simulink model "Target_Control_System"  (R2021b)
settings: Solver=FixedStepDiscrete  StartTime=0.0  StopTime=5  RelTol=1e-3
PreLoadFcn:
  | RTWConfigurationCB('preloadfcn', bdroot);
PostLoadFcn:
  | load('configuration/data_struct.mat');
  | load('configuration/fluxMaps_propMotor.mat');
  | load('configuration/parameterInit_PROP.mat');
  | load('configuration/parameterInit_PUMP.mat');
  | load('configuration/parameterInit_PITCH.mat');
  | load('configuration/parameterInit_TILT.mat');
  | %load('configuration/base_workspace_signal_definition.mat');
  | %load('resolvedatastores_to_baseworkspace_for_faster_simulation.mat');
model workspace (MAT data in the model file):
  SIMULATION_OPTIONS : Simulink.Parameter (value not decoded)
  TARGET_CODE_GEN : Simulink.Parameter (value not decoded)
  TCS_SAMPLE_FREQ_HZ : Simulink.Parameter (value not decoded)
symbols that are objects in the model workspace (value not decoded): TARGET_CODE_GEN, TCS_SAMPLE_FREQ_HZ
undefined symbols (not defined in the file): A_DQ_REF_LPF_INIT__PITCH, A_DQ_REF_LPF_INIT__PROP, A_DQ_REF_LPF_INIT__PUMP, A_DQ_REF_LPF_INIT__TILT, A_OBSERVER_CONFIDENCE_INIT__PITCH, A_OBSERVER_CONFIDENCE_INIT__PROP, A_OBSERVER_CONFIDENCE_INIT__PUMP, A_OBSERVER_CONFIDENCE_INIT__TILT, ACTUATOR_MAX_ANGLE_TRIP__PITCH, ACTUATOR_MIN_ANGLE_TRIP__PITCH, ACTUATOR_POS_SENSOR_INV_DIRECTION__PITCH, ACTUATOR_POS_SENSOR_INV_DIRECTION__TILT, ACTUATOR_POS_SENSOR_OFFSET__PITCH, ACTUATOR_POS_SENSOR_OFFSET__TILT, ADC_scaler1_baseaddr_TILT, ADC_SCALER_FLOAT_TO_FIXPOINT_EXPANSION, ANGLE_ELEC_FROM_SENSOR_OFFSET_INIT__PITCH, ANGLE_ELEC_FROM_SENSOR_OFFSET_INIT__PROP, ANGLE_ELEC_FROM_SENSOR_OFFSET_INIT__PUMP, ANGLE_ELEC_FROM_SENSOR_OFFSET_INIT__TILT, AUTO_CLEAR_FAULTS_ENABLED__PITCH, AUTO_CLEAR_FAULTS_ENABLED__PROP, AUTO_CLEAR_FAULTS_ENABLED__PUMP, AUTO_CLEAR_FAULTS_ENABLED__TILT, AUTO_CLEAR_FAULTS_WAIT_TICKS__PITCH, AUTO_CLEAR_FAULTS_WAIT_TICKS__PROP, AUTO_CLEAR_FAULTS_WAIT_TICKS__PUMP, AUTO_CLEAR_FAULTS_WAIT_TICKS__TILT, AUTO_I_ZERO_IDLE_TICKS__PITCH, AUTO_I_ZERO_IDLE_TICKS__PROP, AUTO_I_ZERO_IDLE_TICKS__PUMP, AUTO_I_ZERO_IDLE_TICKS__TILT, AUTO_I_ZERO_OFFSET_IDC_THRESHOLD__PITCH, AUTO_I_ZERO_OFFSET_IDC_THRESHOLD__PROP, AUTO_I_ZERO_OFFSET_IDC_THRESHOLD__PUMP, AUTO_I_ZERO_OFFSET_IDC_THRESHOLD__TILT, AUTO_I_ZERO_OFFSET_IPH_THRESHOLD__PITCH, AUTO_I_ZERO_OFFSET_IPH_THRESHOLD__PROP, AUTO_I_ZERO_OFFSET_IPH_THRESHOLD__PUMP, AUTO_I_ZERO_OFFSET_IPH_THRESHOLD__TILT, AUTO_SENSORLESS_SWITCHOVER_DISABLE_OMEGA, AUTO_SENSORLESS_SWITCHOVER_ENABLE_OMEGA, AUTO_SENSORLESS_SWITCHOVER_MIN_CONFIDENCE, AUXILIARY_PROTECTION_UNIT_BASEADDR__TILT, blanking_max_error_omega_INIT_PITCH, blanking_max_error_omega_INIT_TILT, blanking_max_error_position_INIT_PITCH, blanking_max_error_position_INIT_TILT, BRUTE_START_I_Q_REF_RAMP_SPEED__PITCH, BRUTE_START_I_Q_REF_RAMP_SPEED__PROP, BRUTE_START_I_Q_REF_RAMP_SPEED__PUMP, BRUTE_START_I_Q_REF_RAMP_SPEED__TILT, CONTROL_LOOP_DT_INIT__PITCH, CONTROL_LOOP_DT_INIT__PROP, CONTROL_LOOP_DT_INIT__PUMP, CONTROL_LOOP_DT_INIT__TILT, CORRECTION_FILTER_SCALE__PITCH, CORRECTION_FILTER_SCALE__PROP, CORRECTION_FILTER_SCALE__PUMP, CORRECTION_FILTER_SCALE__TILT ... (+458)
libraries: simulink x178, Reusables_Lib x24
(part 33 of 47)

== system Target_Control_System/Target_Control_System/MainLoop/pitchMotor_mainLoop/mainTask_pitch/motorTaskMainFastStep()/Control Loops - Pitch/Position Controller Pitch ==
  oRampDataPos_.fRampOut : Inport
  Enable : EnablePort
  Connect PosController to CurrentController : Subsystem
  Data Store Read1 : DataStoreRead  DataStoreName=oPitch  DataStoreElements=oPitch.oMot_.oParam_.fPosition2currentPMultiplier_  IndexOptions=Index vector (dialog)  Indices=1  OutputSizes=1
  Data Store Read10 : DataStoreRead  DataStoreName=oPitch  DataStoreElements=oPitch.oMot_.oState_.oPosSensor_.oPidDataPosCtrl_.oParameter_.fLargeErrorThresholdNegative_  IndexOptions=Index vector (dialog)  Indices=1  OutputSizes=1
  Data Store Read12 : DataStoreRead  DataStoreName=oPitch  DataStoreElements=oPitch.oMot_.oState_.oPosSensor_.oPidDataPosCtrl_.oParameter_.fBlankingMaxError_  IndexOptions=Index vector (dialog)  Indices=1  OutputSizes=1
  Data Store Read14 : DataStoreRead  DataStoreName=oPitch  DataStoreElements=oPitch.oMot_.oState_.oPosSensor_.oPidDataPosCtrl_.oParameter_.fKi_  IndexOptions=Index vector (dialog)  Indices=1  OutputSizes=1
  Data Store Read15 : DataStoreRead  DataStoreName=oPitch  DataStoreElements=oPitch.oMot_.oState_.oPosSensor_.oPidDataPosCtrl_.oParameter_.fLoopDt_  IndexOptions=Index vector (dialog)  Indices=1  OutputSizes=1
  Data Store Read16 : DataStoreRead  DataStoreName=oPitch  DataStoreElements=oPitch.oMot_.oState_.oPosSensor_.oPidDataPosCtrl_.oParameter_.fIntMax_  IndexOptions=Index vector (dialog)  Indices=1  OutputSizes=1
  Data Store Read17 : DataStoreRead  DataStoreName=oPitch  DataStoreElements=oPitch.oMot_.oState_.oPosSensor_.oPidDataPosCtrl_.oParameter_.fIntMin_  IndexOptions=Index vector (dialog)  Indices=1  OutputSizes=1
  Data Store Read18 : DataStoreRead  DataStoreName=oPitch  DataStoreElements=oPitch.oMot_.oState_.oPosSensor_.oPidDataPosCtrl_.oParameter_.ipInhibitTarget_  IndexOptions=Index vector (dialog)  Indices=1  OutputSizes=1
  Data Store Read19 : DataStoreRead  DataStoreName=oPitch  DataStoreElements=oPitch.oMot_.oState_.oPosSensor_.oPidDataPosCtrl_.oParameter_.fIntegratorLeakFactor_  IndexOptions=Index vector (dialog)  Indices=1  OutputSizes=1
  Data Store Read2 : DataStoreRead  DataStoreName=oPitch  DataStoreElements=oPitch.oMot_.oParam_.fPosition2currentIMultiplier_  IndexOptions=Index vector (dialog)  Indices=1  OutputSizes=1
  Data Store Read20 : DataStoreRead  DataStoreName=oPitch  DataStoreElements=oPitch.oMot_.oState_.oPosSensor_.oPidDataPosCtrl_.oParameter_.fKd_  IndexOptions=Index vector (dialog)  Indices=1  OutputSizes=1
  Data Store Read21 : DataStoreRead  DataStoreName=oPitch  DataStoreElements=oPitch.oMot_.oState_.oPosSensor_.oPidDataPosCtrl_.oParameter_.fDMax_  IndexOptions=Index vector (dialog)  Indices=1  OutputSizes=1
  Data Store Read22 : DataStoreRead  DataStoreName=oPitch  DataStoreElements=oPitch.oMot_.oState_.oPosSensor_.oPidDataPosCtrl_.oParameter_.fDMin_  IndexOptions=Index vector (dialog)  Indices=1  OutputSizes=1
  Data Store Read23 : DataStoreRead  DataStoreName=oPitch  DataStoreElements=oPitch.oMot_.oState_.oPosSensor_.oPidDataPosCtrl_.oParameter_.fKp_  IndexOptions=Index vector (dialog)  Indices=1  OutputSizes=1
  Data Store Read24 : DataStoreRead  DataStoreName=oPitch  DataStoreElements=oPitch.oMot_.oState_.oPosSensor_.oPidDataPosCtrl_.oParameter_.fOutMin_  IndexOptions=Index vector (dialog)  Indices=1  OutputSizes=1
  Data Store Read3 : DataStoreRead  DataStoreName=oPitch  DataStoreElements=oPitch.oMot_.oState_.oPosSensor_.oPidDataPosCtrl_.oParameter_.fOutMax_  IndexOptions=Index vector (dialog)  Indices=1  OutputSizes=1
  Data Store Read4 : DataStoreRead  DataStoreName=oPitch  DataStoreElements=oPitch.oMot_.oParam_.fPosition2currentDMultiplier_  IndexOptions=Index vector (dialog)  Indices=1  OutputSizes=1
  Data Store Read5 : DataStoreRead  DataStoreName=oPitch  DataStoreElements=oPitch.oMot_.oState_.oPosSensor_.oGbx_.fCurrentOutputAngle_  IndexOptions=Index vector (dialog)  Indices=1  OutputSizes=1
  Data Store Read6 : DataStoreRead  DataStoreName=oPitch  DataStoreElements=oPitch.oMot_.oState_.oPosSensor_.oPidDataPosCtrl_.fState_  IndexOptions=Index vector (dialog)  Indices=1  OutputSizes=1
  Data Store Read7 : DataStoreRead  DataStoreName=oPitch  DataStoreElements=oPitch.oMot_.oState_.oPosSensor_.fOmegaEFromSensor_  IndexOptions=Index vector (dialog)  Indices=1  OutputSizes=1
  Data Store Read8 : DataStoreRead  DataStoreName=oPitch  DataStoreElements=oPitch.oMot_.oState_.oPosSensor_.oPidDataPosCtrl_.oParameter_.fErrorReduction_  IndexOptions=Index vector (dialog)  Indices=1  OutputSizes=1
  Data Store Read9 : DataStoreRead  DataStoreName=oPitch  DataStoreElements=oPitch.oMot_.oState_.oPosSensor_.oPidDataPosCtrl_.oParameter_.fLargeErrorThresholdPositive_  IndexOptions=Index vector (dialog)  Indices=1  OutputSizes=1
  Data Store Write : DataStoreWrite  DataStoreName=oPitch  DataStoreElements=oPitch.oMot_.oState_.oPosSensor_.oPidDataPosCtrl_.oParameter_.iLargeErrorPresent_  IndexOptions=Index vector (dialog)  Indices=1  OutputSizes=1
  Data Store Write1 : DataStoreWrite  DataStoreName=oPitch  DataStoreElements=oPitch.oMot_.oState_.oPosSensor_.oPidDataPosCtrl_.oParameter_.fITerm_  IndexOptions=Index vector (dialog)  Indices=1  OutputSizes=1
  Data Store Write2 : DataStoreWrite  DataStoreName=oPitch  DataStoreElements=oPitch.oMot_.oState_.oPosSensor_.oPidDataPosCtrl_.oParameter_.fDTerm_  IndexOptions=Index vector (dialog)  Indices=1  OutputSizes=1
  Data Store Write3 : DataStoreWrite  DataStoreName=oPitch  DataStoreElements=oPitch.oMot_.oState_.oPosSensor_.oPidDataPosCtrl_.oParameter_.fPTerm_  IndexOptions=Index vector (dialog)  Indices=1  OutputSizes=1
  Data Store Write4 : DataStoreWrite  DataStoreName=oPitch  DataStoreElements=oPitch.oMot_.oState_.oRampDataOmegaERef_.fSetpoint_  IndexOptions=Index vector (dialog)  Indices=1  OutputSizes=1
  Data Store Write5 : DataStoreWrite  DataStoreName=oPitch  DataStoreElements=oPitch.oMot_.oState_.oPosSensor_.oPidDataPosCtrl_.fState_  IndexOptions=Index vector (dialog)  Indices=1  OutputSizes=1
  Data Store Write6 : DataStoreWrite  DataStoreName=oPitch  DataStoreElements=oPitch.oMot_.oState_.fIqRefFromSpeedController_  IndexOptions=Index vector (dialog)  Indices=1  OutputSizes=1
  pid2ControllerStep(oPidDataPosCtrl)_pitch : Subsystem  TreatAsAtomicUnit=on
  oRampDataOmegaERef_.fSetpoint : Outport
  wires:
  Data Store Read6/1 -> pid2ControllerStep(oPidDataPosCtrl)_pitch/20(fpState)
  Connect PosController to CurrentController/1(fIqRefFromSpeedController) -> Data Store Write6/1
  Data Store Read1/1 -> Connect PosController to CurrentController/2(fIMultiplier)
  Data Store Read2/1 -> Connect PosController to CurrentController/1(fPMultiplier)
  Data Store Read4/1 -> Connect PosController to CurrentController/3(DMultiplier)
  pid2ControllerStep(oPidDataPosCtrl)_pitch/2(fITerm) -> Connect PosController to CurrentController/4(fITerm), Data Store Write1/1
  Data Store Read16/1 -> pid2ControllerStep(oPidDataPosCtrl)_pitch/10(fIntMax)
  pid2ControllerStep(oPidDataPosCtrl)_pitch/4(fPTerm) -> Connect PosController to CurrentController/6(fPTerm), Data Store Write3/1
  Data Store Read20/1 -> pid2ControllerStep(oPidDataPosCtrl)_pitch/13(fKd)
  Data Store Read19/1 -> pid2ControllerStep(oPidDataPosCtrl)_pitch/12(fIntegratorLeakFactor)
  Data Store Read14/1 -> pid2ControllerStep(oPidDataPosCtrl)_pitch/7(fKi)
  Data Store Read15/1 -> pid2ControllerStep(oPidDataPosCtrl)_pitch/9(fLoopDt)
  Data Store Read24/1 -> pid2ControllerStep(oPidDataPosCtrl)_pitch/19(fOutMin)
  pid2ControllerStep(oPidDataPosCtrl)_pitch/3(fDTerm) -> Data Store Write2/1, Connect PosController to CurrentController/5(fDTerm)
  Data Store Read9/1 -> pid2ControllerStep(oPidDataPosCtrl)_pitch/4(fLargeErrorThresholdPositive)
  Data Store Read21/1 -> pid2ControllerStep(oPidDataPosCtrl)_pitch/15(fDMax)
  Data Store Read3/1 -> pid2ControllerStep(oPidDataPosCtrl)_pitch/18(fOutMax)
  Data Store Read17/1 -> pid2ControllerStep(oPidDataPosCtrl)_pitch/11(fIntMin)
  Data Store Read8/1 -> pid2ControllerStep(oPidDataPosCtrl)_pitch/3(fErrorReduction)
  Data Store Read5/1 -> pid2ControllerStep(oPidDataPosCtrl)_pitch/1(fActual)
  pid2ControllerStep(oPidDataPosCtrl)_pitch/1(iLargeErrorPresent) -> Data Store Write/1
  oRampDataPos_.fRampOut/1 -> pid2ControllerStep(oPidDataPosCtrl)_pitch/2(fTarget)
  Data Store Read23/1 -> pid2ControllerStep(oPidDataPosCtrl)_pitch/17(fKp)
  Data Store Read22/1 -> pid2ControllerStep(oPidDataPosCtrl)_pitch/16(fDMin)
  Data Store Read18/1 -> pid2ControllerStep(oPidDataPosCtrl)_pitch/8(ipInhibitTarget)
  pid2ControllerStep(oPidDataPosCtrl)_pitch/5(fOutput) -> Data Store Write4/1, oRampDataOmegaERef_.fSetpoint/1
  Data Store Read12/1 -> pid2ControllerStep(oPidDataPosCtrl)_pitch/6(fBlankingMaxError)
  Data Store Read7/1 -> pid2ControllerStep(oPidDataPosCtrl)_pitch/14(fActualDt)
  pid2ControllerStep(oPidDataPosCtrl)_pitch/6(*fpState) -> Data Store Write5/1
  Data Store Read10/1 -> pid2ControllerStep(oPidDataPosCtrl)_pitch/5(fLargeErrorThresholdNegative)

== system Target_Control_System/Target_Control_System/MainLoop/pitchMotor_mainLoop/mainTask_pitch/motorTaskMainFastStep()/Control Loops - Pitch/Ramp Flux Feedforward ==
  Enable : EnablePort
  Data Store Read19 : DataStoreRead  DataStoreName=oPitch  DataStoreElements=oPitch.oMot_.oState_.oRampDataFluxFeedforwardGain_.oParam_.fTimestepS_  IndexOptions=Index vector (dialog)  Indices=1  OutputSizes=1
  Data Store Read20 : DataStoreRead  DataStoreName=oPitch  DataStoreElements=oPitch.oMot_.oState_.oRampDataFluxFeedforwardGain_.oParam_.fUpslope_  IndexOptions=Index vector (dialog)  Indices=1  OutputSizes=1
  Data Store Read21 : DataStoreRead  DataStoreName=oPitch  DataStoreElements=oPitch.oMot_.oState_.oRampDataFluxFeedforwardGain_.oParam_.fDownslope_  IndexOptions=Index vector (dialog)  Indices=1  OutputSizes=1
  Data Store Read22 : DataStoreRead  DataStoreName=oPitch  DataStoreElements=oPitch.oMot_.oState_.oRampDataFluxFeedforwardGain_.fSetpoint_  IndexOptions=Index vector (dialog)  Indices=1  OutputSizes=1
  Data Store Write10 : DataStoreWrite  DataStoreName=oPitch  DataStoreElements=oPitch.oMot_.oState_.oRampDataFluxFeedforwardGain_.fRampOutDdt_  IndexOptions=Index vector (dialog)  Indices=1  OutputSizes=1
  Data Store Write9 : DataStoreWrite  DataStoreName=oPitch  DataStoreElements=oPitch.oMot_.oState_.oRampDataFluxFeedforwardGain_.fRampOut_  IndexOptions=Index vector (dialog)  Indices=1  OutputSizes=1
  rampStep(oRampDataFluxFeedforwardGain)_pitch : Reusables_Lib/rampStep_  SystemSampleTime=-1  VariantActivationTime=update diagram  Latency=0  AutoFrameSizeCalculation=off
  wires:
  rampStep(oRampDataFluxFeedforwardGain)_pitch/1 -> Data Store Write9/1
  rampStep(oRampDataFluxFeedforwardGain)_pitch/2 -> Data Store Write10/1
  Data Store Read20/1 -> rampStep(oRampDataFluxFeedforwardGain)_pitch/2
  Data Store Read21/1 -> rampStep(oRampDataFluxFeedforwardGain)_pitch/3
  Data Store Read19/1 -> rampStep(oRampDataFluxFeedforwardGain)_pitch/4
  Data Store Read22/1 -> rampStep(oRampDataFluxFeedforwardGain)_pitch/1

== system Target_Control_System/Target_Control_System/MainLoop/pitchMotor_mainLoop/mainTask_pitch/motorTaskMainFastStep()/Control Loops - Pitch/Speed Controller Pitch ==
  oRampDataOmegaERef_.fRampOut : Inport
  Enable : EnablePort
  AND : Logic  AllPortsSameDT=off  OutDataTypeStr=boolean
  Constant : Constant  Value=245  OutDataTypeStr=int32  SampleTime=-1
  Constant1 : Constant  Value=0  OutDataTypeStr=int32  SampleTime=-1
  Data Store Read1 : DataStoreRead  DataStoreName=oPitch  DataStoreElements=oPitch.oMot_.oParam_.uiTorqueMirroringActive_  IndexOptions=Index vector (dialog)  Indices=1  OutputSizes=1
  Data Store Read2 : DataStoreRead  DataStoreName=oPitch  DataStoreElements=oPitch.oMot_.oState_.uiDriveState_  IndexOptions=Index vector (dialog)  Indices=1  OutputSizes=1
  Data Store Read3 : DataStoreRead  DataStoreName=oPitch  DataStoreElements=oPitch.oIsr_.oParam_.iUseSensorAngle_  IndexOptions=Index vector (dialog)  Indices=1  OutputSizes=1
  Enabled Subsystem : Subsystem  TreatAsAtomicUnit=on
  Enabled Subsystem1 : Subsystem  TreatAsAtomicUnit=on
  GreaterThan : RelationalOperator  Operator=>  OutDataTypeStr=boolean  RndMeth=Simplest
  Less Than : RelationalOperator  Operator=<  OutDataTypeStr=boolean  RndMeth=Simplest
  NOT : Logic  Operator=NOT  IconShape=distinctive  AllPortsSameDT=off  OutDataTypeStr=boolean
  NOT1 : Logic  Operator=NOT  AllPortsSameDT=off  OutDataTypeStr=boolean
  Set Iq Ref Pitch : Subsystem  TreatAsAtomicUnit=on
  Switch : Switch  Criteria=u2 > Threshold
  wires:
  Enabled Subsystem1/1(fIqRefFromSpeedController) -> Switch/3
  GreaterThan/1 -> Switch/2, Enabled Subsystem/Enable, NOT1/1
  Constant1/1 -> GreaterThan/2
  Data Store Read3/1 -> GreaterThan/1
  NOT1/1 -> Enabled Subsystem1/Enable
  Switch/1 -> Set Iq Ref Pitch/1(fIqRefFromSpeedController)
  Enabled Subsystem/1(fIqRefFromSpeedController) -> Switch/1
  oRampDataOmegaERef_.fRampOut/1 -> Enabled Subsystem1/1(oRampDataOmegaERef_.fRampOut), Enabled Subsystem/1(oRampDataOmegaERef_.fRampOut)
  Data Store Read2/1 -> Less Than/1
  Data Store Read1/1 -> NOT/1
  Constant/1 -> Less Than/2
  NOT/1 -> AND/1
  Less Than/1 -> AND/2
  AND/1 -> Set Iq Ref Pitch/Enable

== system Target_Control_System/Target_Control_System/MainLoop/pitchMotor_mainLoop/mainTask_pitch/motorTaskMainFastStep()/Correction Constants for Observer and Control - Pitch/1//sqrt(1+u^2) ==
  fTemp : Inport
  Add : Sum
  Constant2 : Constant  OutDataTypeStr=single  SampleTime=-1
  Constant3 : Constant  OutDataTypeStr=single  SampleTime=-1
  Divide5 : Product  Inputs=**
  Divide6 : Product  Inputs=*/
  Sqrt : Sqrt  SaturateOnIntegerOverflow=on
  Out1 : Outport
  wires:
  Divide5/1 -> Add/1
  fTemp/1 -> Divide5/1, Divide5/2
  Add/1 -> Sqrt/1
  Sqrt/1 -> Divide6/2
  Constant3/1 -> Divide6/1
  Constant2/1 -> Add/2
  Divide6/1 -> Out1/1

== system Target_Control_System/Target_Control_System/MainLoop/pitchMotor_mainLoop/mainTask_pitch/motorTaskMainFastStep()/Mechanical System - Pitch/processSensors(&oPitch) ==
  Enable : EnablePort
  Auxiliary sensor : Subsystem
  Data Store Read94 : DataStoreRead  DataStoreName=oPitch  DataStoreElements=oPitch.oMot_.oState_.oPosSensor_.eAuxiliaryPositionSensorType_  IndexOptions=Index vector (dialog)  Indices=1  OutputSizes=1
  Enumerated Constant2 : simulink/Sources/Enumerated Constant  OutDataTypeStr=Enum: EPositionSensor_t  Value=EPositionSensor_t.eNone  SampleTime=-1
  Input (motor) side sensor : Subsystem
  NotEqual : RelationalOperator  Operator=~=  OutDataTypeStr=boolean  RndMeth=Simplest
  Output (actuator) side sensor : Subsystem
  wires:
  NotEqual/1 -> Auxiliary sensor/Enable
  Enumerated Constant2/1 -> NotEqual/2
  Data Store Read94/1 -> NotEqual/1

== system Target_Control_System/Target_Control_System/MainLoop/pitchMotor_mainLoop/mainTask_pitch/motorTaskMainFastStep()/Motor Acceleration - Pitch/First filter stage ==
  function : TriggerPort  TriggerType=function-call  VariantControl=Variant
  Data Store Read : DataStoreRead  DataStoreName=mdl_pitch_fOmegaE  IndexOptions=Index vector (dialog)  Indices=1  OutputSizes=1
  Data Store Read1 : DataStoreRead  DataStoreName=oPitch  DataStoreElements=oPitch.oMot_.oState_.oMotorAccelerationFilterStage1_.afConstantsA_.h0  IndexOptions=Index vector (dialog)  Indices=1  OutputSizes=1
  Data Store Read10 : DataStoreRead  DataStoreName=oPitch  DataStoreElements=oPitch.oMot_.oState_.oMotorAccelerationFilterStage1_.afPreviousOutputs_.h1  IndexOptions=Index vector (dialog)  Indices=1  OutputSizes=1
  Data Store Read11 : DataStoreRead  DataStoreName=oPitch  DataStoreElements=oPitch.oMot_.oState_.fOmegaEPrevious_  IndexOptions=Index vector (dialog)  Indices=1  OutputSizes=1
  Data Store Read2 : DataStoreRead  DataStoreName=oPitch  DataStoreElements=oPitch.oMot_.oState_.oMotorAccelerationFilterStage1_.afConstantsA_.h1  IndexOptions=Index vector (dialog)  Indices=1  OutputSizes=1
  Data Store Read3 : DataStoreRead  DataStoreName=oPitch  DataStoreElements=oPitch.oMot_.oState_.oMotorAccelerationFilterStage1_.afConstantsA_.h2  IndexOptions=Index vector (dialog)  Indices=1  OutputSizes=1
  Data Store Read4 : DataStoreRead  DataStoreName=oPitch  DataStoreElements=oPitch.oMot_.oState_.oMotorAccelerationFilterStage1_.afConstantsB_.h0  IndexOptions=Index vector (dialog)  Indices=1  OutputSizes=1
  Data Store Read5 : DataStoreRead  DataStoreName=oPitch  DataStoreElements=oPitch.oMot_.oState_.oMotorAccelerationFilterStage1_.afConstantsB_.h1  IndexOptions=Index vector (dialog)  Indices=1  OutputSizes=1
  Data Store Read6 : DataStoreRead  DataStoreName=oPitch  DataStoreElements=oPitch.oMot_.oState_.oMotorAccelerationFilterStage1_.afConstantsB_.h2  IndexOptions=Index vector (dialog)  Indices=1  OutputSizes=1
  Data Store Read7 : DataStoreRead  DataStoreName=oPitch  DataStoreElements=oPitch.oMot_.oState_.oMotorAccelerationFilterStage1_.afPreviousInputs_.h0  IndexOptions=Index vector (dialog)  Indices=1  OutputSizes=1
  Data Store Read8 : DataStoreRead  DataStoreName=oPitch  DataStoreElements=oPitch.oMot_.oState_.oMotorAccelerationFilterStage1_.afPreviousInputs_.h1  IndexOptions=Index vector (dialog)  Indices=1  OutputSizes=1
  Data Store Read9 : DataStoreRead  DataStoreName=oPitch  DataStoreElements=oPitch.oMot_.oState_.oMotorAccelerationFilterStage1_.afPreviousOutputs_.h0  IndexOptions=Index vector (dialog)  Indices=1  OutputSizes=1
  Data Store Write1 : DataStoreWrite  DataStoreName=oPitch  DataStoreElements=oPitch.oMot_.oState_.oMotorAccelerationFilterStage1_.fFilterOutput_  IndexOptions=Index vector (dialog)  Indices=1  OutputSizes=1
  Data Store Write2 : DataStoreWrite  DataStoreName=oPitch  DataStoreElements=oPitch.oMot_.oState_.oMotorAccelerationFilterStage1_.afPreviousOutputs_.h0  IndexOptions=Index vector (dialog)  Indices=1  OutputSizes=1
  Data Store Write3 : DataStoreWrite  DataStoreName=oPitch  DataStoreElements=oPitch.oMot_.oState_.oMotorAccelerationFilterStage1_.afPreviousOutputs_.h1  IndexOptions=Index vector (dialog)  Indices=1  OutputSizes=1
  Data Store Write4 : DataStoreWrite  DataStoreName=oPitch  DataStoreElements=oPitch.oMot_.oState_.oMotorAccelerationFilterStage1_.afPreviousInputs_.h0  IndexOptions=Index vector (dialog)  Indices=1  OutputSizes=1
  Data Store Write5 : DataStoreWrite  DataStoreName=oPitch  DataStoreElements=oPitch.oMot_.oState_.oMotorAccelerationFilterStage1_.afPreviousInputs_.h1  IndexOptions=Index vector (dialog)  Indices=1  OutputSizes=1
  Subtract : Sum  Inputs=+-
  softwareIirFilterStep() : Subsystem
  wires:
  softwareIirFilterStep()/3(*afPreviousOutputs1) -> Data Store Write3/1
  Data Store Read3/1 -> softwareIirFilterStep()/7(afConstantsA2)
  Data Store Read11/1 -> Subtract/2
  Subtract/1 -> softwareIirFilterStep()/1(newInput)
  softwareIirFilterStep()/5(fFilterOutput) -> Data Store Write1/1
  Data Store Read6/1 -> softwareIirFilterStep()/4(afConstantsB2)
  Data Store Read8/1 -> softwareIirFilterStep()/9(afPreviousInputs1)
  Data Store Read/1 -> Subtract/1
  Data Store Read7/1 -> softwareIirFilterStep()/8(afPreviousInputs0)
  Data Store Read1/1 -> softwareIirFilterStep()/5(afConstantsA0)
  Data Store Read10/1 -> softwareIirFilterStep()/11(afPreviousOutputs1)
  softwareIirFilterStep()/1(*afPreviousInputs1) -> Data Store Write5/1
  softwareIirFilterStep()/4(*afPreviousOutputs0) -> Data Store Write2/1
  softwareIirFilterStep()/2(*afPreviousInputs0) -> Data Store Write4/1
  Data Store Read2/1 -> softwareIirFilterStep()/6(afConstantsA1)
  Data Store Read9/1 -> softwareIirFilterStep()/10(afPreviousOutputs0)
  Data Store Read5/1 -> softwareIirFilterStep()/3(afConstantsB1)
  Data Store Read4/1 -> softwareIirFilterStep()/2(afConstantsB0)

== system Target_Control_System/Target_Control_System/MainLoop/pitchMotor_mainLoop/mainTask_pitch/motorTaskMainFastStep()/Motor Acceleration - Pitch/Speed step ==
  function : TriggerPort  TriggerType=function-call  VariantControl=Variant
  Data Store Read : DataStoreRead  DataStoreName=mdl_pitch_fOmegaE  IndexOptions=Index vector (dialog)  Indices=1  OutputSizes=1
  Data Store Write : DataStoreWrite  DataStoreName=oPitch  DataStoreElements=oPitch.oMot_.oState_.fOmegaEPrevious_  IndexOptions=Index vector (dialog)  Indices=1  OutputSizes=1
  wires:
  Data Store Read/1 -> Data Store Write/1

== system Target_Control_System/Target_Control_System/MainLoop/pitchMotor_mainLoop/mainTask_pitch/motorTaskMainFastStep()/Observer Confidence - Pitch/Automatic switching to sensorless ==
  In1 : Inport
  Enable : EnablePort
  Data Store Read27 : DataStoreRead  DataStoreName=oPitch  DataStoreElements=oPitch.oMot_.oState_.uiSensorlessSwitchoverState_  IndexOptions=Index vector (dialog)  Indices=1  OutputSizes=1
  If : If
  "Switch to sensored? " : Subsystem  TreatAsAtomicUnit=on
  Switch to sensorless? : Subsystem  TreatAsAtomicUnit=on
  wires:
  In1/1 -> "Switch to sensored? "/1(fObserverConfidence), Switch to sensorless?/1(fObserverConfidence)
  Data Store Read27/1 -> If/1
  If/1 -> "Switch to sensored? "/Action
  If/2 -> Switch to sensorless?/Action

== system Target_Control_System/Target_Control_System/MainLoop/pitchMotor_mainLoop/mainTask_pitch/motorTaskMainFastStep()/Observer Confidence - Pitch/IIR ==
  In : Inport
  1-K : Inport  Port=2
  K : Inport  Port=3
  Product : Product  OutDataTypeStr=single  RndMeth=Zero
  Product1 : Product  RndMeth=Zero
  Sum : Sum  Inputs=|++  OutDataTypeStr=single
  Unit Delay : UnitDelay  SampleTime=-1  HasFrameUpgradeWarning=on
  Out : Outport
  wires:
  Sum/1 -> Unit Delay/1, Out/1
  Unit Delay/1 -> Product/1
  K/1 -> Product1/2
  1-K/1 -> Product/2
  Product/1 -> Sum/1
  Product1/1 -> Sum/2
  In/1 -> Product1/1

== system Target_Control_System/Target_Control_System/MainLoop/pitchMotor_mainLoop/mainTask_pitch/motorTaskMainFastStep()/Software Overcurrent Protection - Pitch/Forced_angle_overcurrent ==
  Enable : EnablePort
  Chart : Stateflow chart  TreatAsAtomicUnit=on

== system Target_Control_System/Target_Control_System/MainLoop/pitchMotor_mainLoop/mainTask_pitch/motorTaskMainFastStep()/Software Overcurrent Protection - Pitch/checkForHwOvercurrents(&oPitch) ==
  Enable : EnablePort
  "checkForHwOvercurrents " : Stateflow chart  TreatAsAtomicUnit=on
  gateDriverStatus : Subsystem  Variant=on

== system Target_Control_System/Target_Control_System/MainLoop/propMotor_mainLoop/Decimation gate for 5000 Hz Prop/motorTaskProcessExternalSetpoints(&oProp)/Subsystem1/Subsystem ==
  Enable : EnablePort
  Data Store Read68 : DataStoreRead  DataStoreName=oProp  DataStoreElements=oProp.oMot_.oParam_.fDynILimDynamicMax_  IndexOptions=Index vector (dialog)  Indices=1  OutputSizes=1
  Data Store Write19 : DataStoreWrite  DataStoreName=oProp  DataStoreElements=oProp.oMot_.oIn_.fIqSetpoint_  IndexOptions=Index vector (dialog)  Indices=1  OutputSizes=1
  wires:
  Data Store Read68/1 -> Data Store Write19/1

== system Target_Control_System/Target_Control_System/MainLoop/propMotor_mainLoop/Decimation gate for 5000 Hz Prop/motorTaskProcessExternalSetpoints(&oProp)/Subsystem2/Subsystem ==
  Enable : EnablePort
  Data Store Write19 : DataStoreWrite  DataStoreName=oProp  DataStoreElements=oProp.oMot_.oIn_.fIqSetpoint_  IndexOptions=Index vector (dialog)  Indices=1  OutputSizes=1
  const1 : Constant  Value=0.0  OutDataTypeStr=single  SampleTime=-1
  wires:
  const1/1 -> Data Store Write19/1

== system Target_Control_System/Target_Control_System/MainLoop/propMotor_mainLoop/Decimation gate for 5000 Hz Prop/motorTaskProcessExternalSetpoints(&oProp)/Subsystem3/Subsystem ==
  Enable : EnablePort
  AND : Logic  AllPortsSameDT=off  OutDataTypeStr=boolean
  AND1 : Logic  AllPortsSameDT=off  OutDataTypeStr=boolean
  Data Store Read1 : DataStoreRead  DataStoreName=oProp  DataStoreElements=oProp.oMot_.oState_.uiSpeedControllerActive_  IndexOptions=Index vector (dialog)  Indices=1  OutputSizes=1
  Data Store Read2 : DataStoreRead  DataStoreName=oProp  DataStoreElements=oProp.oMot_.oState_.oPosSensor_.iPosControlEnabled_  IndexOptions=Index vector (dialog)  Indices=1  OutputSizes=1
  Data Store Read68 : DataStoreRead  DataStoreName=oProp  DataStoreElements=oProp.oMot_.oIn_.fIqSetpoint_  IndexOptions=Index vector (dialog)  Indices=1  OutputSizes=1
  Data Store Read85 : DataStoreRead  DataStoreName=oProp  DataStoreElements=oProp.oMot_.oParam_.uiTorqueMirroringActive_  IndexOptions=Index vector (dialog)  Indices=1  OutputSizes=1
  IsNaN : RelationalOperator  Operator=isNaN  OutDataTypeStr=boolean  RndMeth=Simplest
  NOT : Logic  Operator=NOT  AllPortsSameDT=off  OutDataTypeStr=boolean
  NOT1 : Logic  Operator=NOT  AllPortsSameDT=off  OutDataTypeStr=boolean
  NOT2 : Logic  Operator=NOT  AllPortsSameDT=off  OutDataTypeStr=boolean
  OR : Logic  Operator=OR  AllPortsSameDT=off  OutDataTypeStr=boolean
  Subsystem : Subsystem
  wires:
  AND1/1 -> Subsystem/Enable
  Data Store Read85/1 -> OR/1
  Data Store Read1/1 -> NOT/1
  AND/1 -> OR/2
  NOT/1 -> AND/1
  Data Store Read2/1 -> NOT1/1
  NOT1/1 -> AND/2
  OR/1 -> AND1/1
  Data Store Read68/1 -> IsNaN/1
  IsNaN/1 -> NOT2/1
  NOT2/1 -> AND1/2

== system Target_Control_System/Target_Control_System/MainLoop/propMotor_mainLoop/Decimation gate for 5000 Hz Prop/motorTaskProcessExternalSetpoints(&oProp)/Subsystem3/Subsystem1 ==
  Enable : EnablePort
  AND1 : Logic  Operator=OR  AllPortsSameDT=off  OutDataTypeStr=boolean
  Data Store Read1 : DataStoreRead  DataStoreName=oProp  DataStoreElements=oProp.oMot_.oIn_.fIdSetpoint_  IndexOptions=Index vector (dialog)  Indices=1  OutputSizes=1
  IsNaN : RelationalOperator  Operator=isNaN  OutDataTypeStr=boolean  RndMeth=Simplest
  IsNaN1 : RelationalOperator  Operator=isInf  OutDataTypeStr=boolean  RndMeth=Simplest
  NOT1 : Logic  Operator=NOT  AllPortsSameDT=off  OutDataTypeStr=boolean
  Subsystem : Subsystem
  wires:
  NOT1/1 -> AND1/1
  Data Store Read1/1 -> IsNaN1/1, Subsystem/1(Input), IsNaN/1
  IsNaN1/1 -> AND1/2
  IsNaN/1 -> NOT1/1
  AND1/1 -> Subsystem/Enable

== system Target_Control_System/Target_Control_System/MainLoop/propMotor_mainLoop/Decimation gate for 5000 Hz Prop/motorTaskProcessExternalSetpoints(&oProp)/Subsystem3/Subsystem2 ==
  Enable : EnablePort
  AND1 : Logic  Inputs=3  AllPortsSameDT=off  OutDataTypeStr=boolean
  Data Store Read1 : DataStoreRead  DataStoreName=oProp  DataStoreElements=oProp.oMot_.oState_.oPosSensor_.iPosControlEnabled_  IndexOptions=Index vector (dialog)  Indices=1  OutputSizes=1
  Data Store Read2 : DataStoreRead  DataStoreName=oProp  DataStoreElements=oProp.oMot_.oParam_.uiAutomaticFanControlMode_  IndexOptions=Index vector (dialog)  Indices=1  OutputSizes=1
  Data Store Read85 : DataStoreRead  DataStoreName=oProp  DataStoreElements=oProp.oMot_.oState_.uiDriveState_  IndexOptions=Index vector (dialog)  Indices=1  OutputSizes=1
  Equal13 : RelationalOperator  Operator=~=  OutDataTypeStr=boolean  RndMeth=Simplest
  NOT1 : Logic  Operator=NOT  AllPortsSameDT=off  OutDataTypeStr=boolean
  NOT2 : Logic  Operator=NOT  AllPortsSameDT=off  OutDataTypeStr=boolean
  Subsystem : Subsystem
  const17 : Constant  Value=228  OutDataTypeStr=uint32  SampleTime=-1
  wires:
  Data Store Read2/1 -> NOT2/1
  NOT2/1 -> AND1/2
  const17/1 -> Equal13/1
  Data Store Read85/1 -> Equal13/2
  Equal13/1 -> AND1/3
  NOT1/1 -> AND1/1
  Data Store Read1/1 -> NOT1/1
  AND1/1 -> Subsystem/Enable

== system Target_Control_System/Target_Control_System/MainLoop/propMotor_mainLoop/Decimation gate for 5000 Hz Prop/motorTaskProcessExternalSetpoints(&oProp)/Subsystem3/Subsystem3 ==
  Enable : EnablePort
  AND : Logic  Operator=OR  AllPortsSameDT=off  OutDataTypeStr=boolean
  AND1 : Logic  Inputs=3  AllPortsSameDT=off  OutDataTypeStr=boolean
  Data Store Read1 : DataStoreRead  DataStoreName=oProp  DataStoreElements=oProp.oMot_.oState_.oPosSensor_.iPosControlEnabled_  IndexOptions=Index vector (dialog)  Indices=1  OutputSizes=1
  Data Store Read68 : DataStoreRead  DataStoreName=oProp  DataStoreElements=oProp.oMot_.oIn_.fPosSetpoint_  IndexOptions=Index vector (dialog)  Indices=1  OutputSizes=1
  Data Store Read85 : DataStoreRead  DataStoreName=oProp  DataStoreElements=oProp.oMot_.oState_.uiDriveState_  IndexOptions=Index vector (dialog)  Indices=1  OutputSizes=1
  Equal1 : RelationalOperator  Operator=~=  OutDataTypeStr=boolean  RndMeth=Simplest
  Equal13 : RelationalOperator  Operator===  OutDataTypeStr=boolean  RndMeth=Simplest
  IsNaN : RelationalOperator  Operator=isNaN  OutDataTypeStr=boolean  RndMeth=Simplest
  NOT2 : Logic  Operator=NOT  AllPortsSameDT=off  OutDataTypeStr=boolean
  Subsystem : Subsystem
  const1 : Constant  Value=202  OutDataTypeStr=uint32  SampleTime=-1
  const17 : Constant  Value=228  OutDataTypeStr=uint32  SampleTime=-1
  wires:
  NOT2/1 -> AND1/3
  const1/1 -> Equal1/2
  Equal1/1 -> AND1/2
  const17/1 -> Equal13/1
  Data Store Read85/1 -> Equal1/1, Equal13/2
  Equal13/1 -> AND/2
  AND/1 -> AND1/1
  Data Store Read1/1 -> AND/1
  IsNaN/1 -> NOT2/1
  Data Store Read68/1 -> IsNaN/1
  AND1/1 -> Subsystem/Enable

== system Target_Control_System/Target_Control_System/MainLoop/propMotor_mainLoop/Decimation gate for 5000 Hz Prop/motorTaskProcessExternalSetpoints(&oProp)/Subsystem3/Subsystem4 ==
  Enable : EnablePort
  Data Store Write1 : DataStoreWrite  DataStoreName=oProp  DataStoreElements=oProp.oMot_.oState_.fIdExternalSetpoint_  IndexOptions=Index vector (dialog)  Indices=1  OutputSizes=1
  Data Store Write19 : DataStoreWrite  DataStoreName=oProp  DataStoreElements=oProp.oMot_.oState_.oRampDataIdRef_.fSetpoint_  IndexOptions=Index vector (dialog)  Indices=1  OutputSizes=1
  const1 : Constant  Value=0.0  OutDataTypeStr=single  SampleTime=-1
  wires:
  const1/1 -> Data Store Write19/1, Data Store Write1/1

== system Target_Control_System/Target_Control_System/MainLoop/propMotor_mainLoop/motorTaskMainFastStep(&oProp)/Control Loops - Prop/Sim Options Prop Id Variant Subsystem/Sim Options 0 Prop Id Subsystem ==
  Data Store Read1 : DataStoreRead  DataStoreName=oProp  DataStoreElements=oProp.oMot_.oState_.oRampDataIdRef_.fSetpoint_  IndexOptions=Index vector (dialog)  Indices=1  OutputSizes=1
  Scope : Scope
  Out1 : Outport
  wires:
  Data Store Read1/1 -> Out1/1, Scope/1

== system Target_Control_System/Target_Control_System/MainLoop/propMotor_mainLoop/motorTaskMainFastStep(&oProp)/Control Loops - Prop/Sim Options Prop Id Variant Subsystem/Sim Options 1 Prop Iq Subsystem ==
  Constant : Constant  Value=0  OutDataTypeStr=single  SampleTime=-1
  Constant1 : Constant  OutDataTypeStr=uint32  SampleTime=-1
  Data Store Write : DataStoreWrite  DataStoreName=oProp  DataStoreElements=oProp.oMot_.oState_.oRampDataIdRef_.fSetpoint_  IndexOptions=Index vector (dialog)  Indices=1  OutputSizes=1
  Data Store Write2 : DataStoreWrite  DataStoreName=oProp  DataStoreElements=oProp.oMot_.oOut_.uiCurrentControllerActive_  IndexOptions=Index vector (dialog)  Indices=1  OutputSizes=1
  Out1 : Outport
  wires:
  Constant1/1 -> Data Store Write2/1
  Constant/1 -> Out1/1, Data Store Write/1

== system Target_Control_System/Target_Control_System/MainLoop/propMotor_mainLoop/motorTaskMainFastStep(&oProp)/Control Loops - Prop/Sim Options Prop Iq Variant Subsystem/Sim Options 0 Prop Iq Subsystem ==
  Data Store Read1 : DataStoreRead  DataStoreName=oProp  DataStoreElements=oProp.oMot_.oState_.oRampDataIqRef_.fSetpoint_  IndexOptions=Index vector (dialog)  Indices=1  OutputSizes=1
  Scope : Scope
  Out1 : Outport
  wires:
  Data Store Read1/1 -> Out1/1, Scope/1

== system Target_Control_System/Target_Control_System/MainLoop/propMotor_mainLoop/motorTaskMainFastStep(&oProp)/Control Loops - Prop/Sim Options Prop Iq Variant Subsystem/Sim Options 1 Prop Iq Subsystem ==
  Constant : Constant  Value=300  OutDataTypeStr=single
  Constant1 : Constant  OutDataTypeStr=uint32  SampleTime=-1
  Data Store Write : DataStoreWrite  DataStoreName=oProp  DataStoreElements=oProp.oMot_.oState_.oRampDataIqRef_.fSetpoint_  IndexOptions=Index vector (dialog)  Indices=1  OutputSizes=1
  Data Store Write2 : DataStoreWrite  DataStoreName=oProp  DataStoreElements=oProp.oMot_.oOut_.uiCurrentControllerActive_  IndexOptions=Index vector (dialog)  Indices=1  OutputSizes=1
  Out1 : Outport
  wires:
  Constant1/1 -> Data Store Write2/1
  Constant/1 -> Out1/1, Data Store Write/1

== system Target_Control_System/Target_Control_System/MainLoop/propMotor_mainLoop/motorTaskMainFastStep(&oProp)/Control Loops - Prop/Subsystem2/Subsystem ==
  fFluxWeakeningModulationTarget_ : Inport
  fModulationIndexSquared : Inport  Port=2
  fFluxWeakeningState_ : Inport  Port=3
  fIntControlLoopDt_ : Inport  Port=4
  Enable : EnablePort
  Add : Sum  Inputs=|++
  Add3 : Sum  Inputs=-+
  Constant4 : Constant  Value=0  OutDataTypeStr=single  SampleTime=-1
  Data Store Read94 : DataStoreRead  DataStoreName=oProp  DataStoreElements=oProp.oMot_.oParam_.fFluxWeakeningUpRampGain_  IndexOptions=Index vector (dialog)  Indices=1  OutputSizes=1
  Data Store Read96 : DataStoreRead  DataStoreName=oProp  DataStoreElements=oProp.oMot_.oParam_.fFluxWeakeningMaxCurrent_  IndexOptions=Index vector (dialog)  Indices=1  OutputSizes=1
  Display : Display
  Product : Product
  Product3 : Product
  Saturation Dynamic : simulink/Discontinuities/Saturation Dynamic  OutMin=[]  OutMax=[]  OutDataTypeStr=Inherit: Same as second input  OutDataType=fixdt(1, 16)  OutScaling=2^-10  DoSatur=off
  Out1 : Outport
  wires:
  Constant4/1 -> Saturation Dynamic/3
  Add/1 -> Saturation Dynamic/2
  Product/1 -> Add/1
  Product3/1 -> Product/1
  fIntControlLoopDt_/1 -> Product/2
  fFluxWeakeningState_/1 -> Add/2
  Data Store Read96/1 -> Display/1, Saturation Dynamic/1
  Add3/1 -> Product3/1  "fDelta"
  fFluxWeakeningModulationTarget_/1 -> Add3/1
  fModulationIndexSquared/1 -> Add3/2
  Saturation Dynamic/1 -> Out1/1
  Data Store Read94/1 -> Product3/2

== system Target_Control_System/Target_Control_System/MainLoop/propMotor_mainLoop/motorTaskMainFastStep(&oProp)/Control Loops - Prop/Subsystem2/Subsystem1 ==
  fFluxWeakeningDownRamp_ : Inport
  fIntControlLoopDt_ : Inport  Port=2
  fFluxWeakeningState_ : Inport  Port=3
  Enable : EnablePort
  Add13 : Sum  Inputs=-+
  Constant4 : Constant  Value=0  OutDataTypeStr=single  SampleTime=-1
  Product2 : Product
  Switch9 : Switch  Criteria=u2 > Threshold
  Out1 : Outport
  wires:
  Constant4/1 -> Switch9/3
  Add13/1 -> Switch9/1
  Switch9/1 -> Out1/1
  fFluxWeakeningState_/1 -> Add13/2, Switch9/2
  fFluxWeakeningDownRamp_/1 -> Product2/1
  Product2/1 -> Add13/1
  fIntControlLoopDt_/1 -> Product2/2

== system Target_Control_System/Target_Control_System/MainLoop/propMotor_mainLoop/motorTaskMainFastStep(&oProp)/Correction Constants for Observer and Control - Prop/Variant Subsystem/Simulation Subsystem ==
  In1 : Inport
  Gain6 : Gain  Gain=1/(6000*2*pi)
  Out1 : Outport
  wires:
  Gain6/1 -> Out1/1
  In1/1 -> Gain6/1

== system Target_Control_System/Target_Control_System/MainLoop/propMotor_mainLoop/motorTaskMainFastStep(&oProp)/Correction Constants for Observer and Control - Prop/Variant Subsystem/Target Code Gen Subsystem ==
  In1 : Inport
  Data Store Read9 : DataStoreRead  DataStoreName=oProp  DataStoreElements=oProp.oMot_.oParam_.fUphaseIirFLpfRads_  IndexOptions=Index vector (dialog)  Indices=1  OutputSizes=1
  Divide2 : Product  Inputs=*/
  Out1 : Outport
  wires:
  In1/1 -> Divide2/1
  Data Store Read9/1 -> Divide2/2
  Divide2/1 -> Out1/1

== system Target_Control_System/Target_Control_System/MainLoop/propMotor_mainLoop/motorTaskMainFastStep(&oProp)/PWM for Simulation/Subsystem1/Subsystem ==
  Enable : EnablePort
  Bus Creator2 : BusCreator  Inputs=3
  Data Store Read2 : DataStoreRead  DataStoreName=oProp  DataStoreElements=oProp.oMot_.oOut_.uiPwmDutyTicksFromMainA_  IndexOptions=Index vector (dialog)  Indices=1  OutputSizes=1
  Data Store Read3 : DataStoreRead  DataStoreName=oProp  DataStoreElements=oProp.oMot_.oOut_.uiPwmDutyTicksFromMainB_  IndexOptions=Index vector (dialog)  Indices=1  OutputSizes=1
  Data Store Read5 : DataStoreRead  DataStoreName=oProp  DataStoreElements=oProp.oMot_.oOut_.uiPwmDutyTicksFromMainC_  IndexOptions=Index vector (dialog)  Indices=1  OutputSizes=1
  propMotor_PWMticks : Outport
  wires:
  Data Store Read3/1 -> Bus Creator2/2  "Bticks"
  Data Store Read5/1 -> Bus Creator2/3  "Cticks"
  Bus Creator2/1 -> propMotor_PWMticks/1
  Data Store Read2/1 -> Bus Creator2/1  "Aticks"

== system Target_Control_System/Target_Control_System/MainLoop/pumpMotor_mainLoop/Decimation gate for 5000 Hz Pump/motorTaskProcessExternalSetpoints(&oPump)/Subsystem1/Subsystem ==
  Enable : EnablePort
  Data Store Read68 : DataStoreRead  DataStoreName=oPump  DataStoreElements=oPump.oMot_.oParam_.fDynILimDynamicMax_  IndexOptions=Index vector (dialog)  Indices=1  OutputSizes=1
  Data Store Write19 : DataStoreWrite  DataStoreName=oPump  DataStoreElements=oPump.oMot_.oIn_.fIqSetpoint_  IndexOptions=Index vector (dialog)  Indices=1  OutputSizes=1
  wires:
  Data Store Read68/1 -> Data Store Write19/1

== system Target_Control_System/Target_Control_System/MainLoop/pumpMotor_mainLoop/Decimation gate for 5000 Hz Pump/motorTaskProcessExternalSetpoints(&oPump)/Subsystem2/Subsystem ==
  Enable : EnablePort
  Data Store Write19 : DataStoreWrite  DataStoreName=oPump  DataStoreElements=oPump.oMot_.oIn_.fIqSetpoint_  IndexOptions=Index vector (dialog)  Indices=1  OutputSizes=1
  const1 : Constant  Value=0.0  OutDataTypeStr=single  SampleTime=-1
  wires:
  const1/1 -> Data Store Write19/1

== system Target_Control_System/Target_Control_System/MainLoop/pumpMotor_mainLoop/Decimation gate for 5000 Hz Pump/motorTaskProcessExternalSetpoints(&oPump)/Subsystem3/Subsystem ==
  Enable : EnablePort
  AND : Logic  AllPortsSameDT=off  OutDataTypeStr=boolean
  AND1 : Logic  AllPortsSameDT=off  OutDataTypeStr=boolean
  Data Store Read1 : DataStoreRead  DataStoreName=oPump  DataStoreElements=oPump.oMot_.oState_.uiSpeedControllerActive_  IndexOptions=Index vector (dialog)  Indices=1  OutputSizes=1
  Data Store Read2 : DataStoreRead  DataStoreName=oPump  DataStoreElements=oPump.oMot_.oState_.oPosSensor_.iPosControlEnabled_  IndexOptions=Index vector (dialog)  Indices=1  OutputSizes=1
  Data Store Read68 : DataStoreRead  DataStoreName=oPump  DataStoreElements=oPump.oMot_.oIn_.fIqSetpoint_  IndexOptions=Index vector (dialog)  Indices=1  OutputSizes=1
  Data Store Read85 : DataStoreRead  DataStoreName=oPump  DataStoreElements=oPump.oMot_.oParam_.uiTorqueMirroringActive_  IndexOptions=Index vector (dialog)  Indices=1  OutputSizes=1
  IsNaN : RelationalOperator  Operator=isNaN  OutDataTypeStr=boolean  RndMeth=Simplest
  NOT : Logic  Operator=NOT  AllPortsSameDT=off  OutDataTypeStr=boolean
  NOT1 : Logic  Operator=NOT  AllPortsSameDT=off  OutDataTypeStr=boolean
  NOT2 : Logic  Operator=NOT  AllPortsSameDT=off  OutDataTypeStr=boolean
  OR : Logic  Operator=OR  AllPortsSameDT=off  OutDataTypeStr=boolean
  Subsystem : Subsystem
  wires:
  AND1/1 -> Subsystem/Enable
  Data Store Read85/1 -> OR/1
  Data Store Read1/1 -> NOT/1
  AND/1 -> OR/2
  NOT/1 -> AND/1
  Data Store Read2/1 -> NOT1/1
  NOT1/1 -> AND/2
  OR/1 -> AND1/1
  Data Store Read68/1 -> IsNaN/1
  IsNaN/1 -> NOT2/1
  NOT2/1 -> AND1/2

== system Target_Control_System/Target_Control_System/MainLoop/pumpMotor_mainLoop/Decimation gate for 5000 Hz Pump/motorTaskProcessExternalSetpoints(&oPump)/Subsystem3/Subsystem1 ==
  Enable : EnablePort
  AND1 : Logic  Operator=OR  AllPortsSameDT=off  OutDataTypeStr=boolean
  Data Store Read1 : DataStoreRead  DataStoreName=oPump  DataStoreElements=oPump.oMot_.oIn_.fIdSetpoint_  IndexOptions=Index vector (dialog)  Indices=1  OutputSizes=1
  IsNaN : RelationalOperator  Operator=isNaN  OutDataTypeStr=boolean  RndMeth=Simplest
  IsNaN1 : RelationalOperator  Operator=isInf  OutDataTypeStr=boolean  RndMeth=Simplest
  NOT1 : Logic  Operator=NOT  AllPortsSameDT=off  OutDataTypeStr=boolean
  Subsystem : Subsystem
  wires:
  NOT1/1 -> AND1/1
  Data Store Read1/1 -> IsNaN1/1, Subsystem/1(Input), IsNaN/1
  IsNaN1/1 -> AND1/2
  IsNaN/1 -> NOT1/1
  AND1/1 -> Subsystem/Enable

== system Target_Control_System/Target_Control_System/MainLoop/pumpMotor_mainLoop/Decimation gate for 5000 Hz Pump/motorTaskProcessExternalSetpoints(&oPump)/Subsystem3/Subsystem2 ==
  Enable : EnablePort
  AND1 : Logic  Inputs=3  AllPortsSameDT=off  OutDataTypeStr=boolean
  Data Store Read1 : DataStoreRead  DataStoreName=oPump  DataStoreElements=oPump.oMot_.oState_.oPosSensor_.iPosControlEnabled_  IndexOptions=Index vector (dialog)  Indices=1  OutputSizes=1
  Data Store Read2 : DataStoreRead  DataStoreName=oPump  DataStoreElements=oPump.oMot_.oParam_.uiAutomaticFanControlMode_  IndexOptions=Index vector (dialog)  Indices=1  OutputSizes=1
  Data Store Read85 : DataStoreRead  DataStoreName=oPump  DataStoreElements=oPump.oMot_.oState_.uiDriveState_  IndexOptions=Index vector (dialog)  Indices=1  OutputSizes=1
  Equal13 : RelationalOperator  Operator=~=  OutDataTypeStr=boolean  RndMeth=Simplest
  NOT1 : Logic  Operator=NOT  AllPortsSameDT=off  OutDataTypeStr=boolean
  NOT2 : Logic  Operator=NOT  AllPortsSameDT=off  OutDataTypeStr=boolean
  Subsystem : Subsystem
  const17 : Constant  Value=228  OutDataTypeStr=uint32  SampleTime=-1
  wires:
  Data Store Read2/1 -> NOT2/1
  NOT2/1 -> AND1/2
  const17/1 -> Equal13/1
  Data Store Read85/1 -> Equal13/2
  Equal13/1 -> AND1/3
  NOT1/1 -> AND1/1
  Data Store Read1/1 -> NOT1/1
  AND1/1 -> Subsystem/Enable

== system Target_Control_System/Target_Control_System/MainLoop/pumpMotor_mainLoop/Decimation gate for 5000 Hz Pump/motorTaskProcessExternalSetpoints(&oPump)/Subsystem3/Subsystem3 ==
  Enable : EnablePort
  AND : Logic  Operator=OR  AllPortsSameDT=off  OutDataTypeStr=boolean
  AND1 : Logic  Inputs=3  AllPortsSameDT=off  OutDataTypeStr=boolean
  Data Store Read1 : DataStoreRead  DataStoreName=oPump  DataStoreElements=oPump.oMot_.oState_.oPosSensor_.iPosControlEnabled_  IndexOptions=Index vector (dialog)  Indices=1  OutputSizes=1
  Data Store Read68 : DataStoreRead  DataStoreName=oPump  DataStoreElements=oPump.oMot_.oIn_.fPosSetpoint_  IndexOptions=Index vector (dialog)  Indices=1  OutputSizes=1
  Data Store Read85 : DataStoreRead  DataStoreName=oPump  DataStoreElements=oPump.oMot_.oState_.uiDriveState_  IndexOptions=Index vector (dialog)  Indices=1  OutputSizes=1
  Equal1 : RelationalOperator  Operator=~=  OutDataTypeStr=boolean  RndMeth=Simplest
  Equal13 : RelationalOperator  Operator===  OutDataTypeStr=boolean  RndMeth=Simplest
  IsNaN : RelationalOperator  Operator=isNaN  OutDataTypeStr=boolean  RndMeth=Simplest
  NOT2 : Logic  Operator=NOT  AllPortsSameDT=off  OutDataTypeStr=boolean
  Subsystem : Subsystem
  const1 : Constant  Value=202  OutDataTypeStr=uint32  SampleTime=-1
  const17 : Constant  Value=228  OutDataTypeStr=uint32  SampleTime=-1
  wires:
  NOT2/1 -> AND1/3
  const1/1 -> Equal1/2
  Equal1/1 -> AND1/2
  const17/1 -> Equal13/1
  Data Store Read85/1 -> Equal1/1, Equal13/2
  Equal13/1 -> AND/2
  AND/1 -> AND1/1
  Data Store Read1/1 -> AND/1
  IsNaN/1 -> NOT2/1
  Data Store Read68/1 -> IsNaN/1
  AND1/1 -> Subsystem/Enable

== system Target_Control_System/Target_Control_System/MainLoop/pumpMotor_mainLoop/Decimation gate for 5000 Hz Pump/motorTaskProcessExternalSetpoints(&oPump)/Subsystem3/Subsystem4 ==
  Enable : EnablePort
  Data Store Write1 : DataStoreWrite  DataStoreName=oPump  DataStoreElements=oPump.oMot_.oState_.fIdExternalSetpoint_  IndexOptions=Index vector (dialog)  Indices=1  OutputSizes=1
  Data Store Write19 : DataStoreWrite  DataStoreName=oPump  DataStoreElements=oPump.oMot_.oState_.oRampDataIdRef_.fSetpoint_  IndexOptions=Index vector (dialog)  Indices=1  OutputSizes=1
  const1 : Constant  Value=0.0  OutDataTypeStr=single  SampleTime=-1
  wires:
  const1/1 -> Data Store Write19/1, Data Store Write1/1

== system Target_Control_System/Target_Control_System/MainLoop/pumpMotor_mainLoop/motorTaskMainFastStep(&oPump)/Control Loops - Pump/Sim Options Prop Id Variant Subsystem/Sim Options 0 Prop Id Subsystem ==
  Data Store Read88 : DataStoreRead  DataStoreName=oPump  DataStoreElements=oPump.oMot_.oState_.oRampDataIdRef_.fSetpoint_  IndexOptions=Index vector (dialog)  Indices=1  OutputSizes=1
  Out1 : Outport
  wires:
  Data Store Read88/1 -> Out1/1

== system Target_Control_System/Target_Control_System/MainLoop/pumpMotor_mainLoop/motorTaskMainFastStep(&oPump)/Control Loops - Pump/Sim Options Prop Id Variant Subsystem/Sim Options 1 Prop Id Subsystem ==
  Constant : Constant  Value=0  OutDataTypeStr=single  SampleTime=-1
  Constant1 : Constant  OutDataTypeStr=uint32  SampleTime=-1
  Data Store Write : DataStoreWrite  DataStoreName=oPump  DataStoreElements=oPump.oMot_.oState_.oRampDataIdRef_.fSetpoint_  IndexOptions=Index vector (dialog)  Indices=1  OutputSizes=1
  Data Store Write2 : DataStoreWrite  DataStoreName=oPump  DataStoreElements=oPump.oMot_.oOut_.uiCurrentControllerActive_  IndexOptions=Index vector (dialog)  Indices=1  OutputSizes=1
  Out1 : Outport
  wires:
  Constant1/1 -> Data Store Write2/1
  Constant/1 -> Out1/1, Data Store Write/1

== system Target_Control_System/Target_Control_System/MainLoop/pumpMotor_mainLoop/motorTaskMainFastStep(&oPump)/Control Loops - Pump/Sim Options Pump Iq Variant Subsystem/Sim Options 0 Pump Iq Subsystem ==
  Data Store Read88 : DataStoreRead  DataStoreName=oPump  DataStoreElements=oPump.oMot_.oState_.oRampDataIqRef_.fSetpoint_  IndexOptions=Index vector (dialog)  Indices=1  OutputSizes=1
  fSetpoint_ : Outport
  wires:
  Data Store Read88/1 -> fSetpoint_/1

== system Target_Control_System/Target_Control_System/MainLoop/pumpMotor_mainLoop/motorTaskMainFastStep(&oPump)/Control Loops - Pump/Sim Options Pump Iq Variant Subsystem/Sim Options 1 Pump Iq Subsystem ==
  Constant : Constant  Value=1.5  OutDataTypeStr=single
  Constant1 : Constant  OutDataTypeStr=uint32  SampleTime=-1
  Data Store Write : DataStoreWrite  DataStoreName=oPump  DataStoreElements=oPump.oMot_.oState_.oRampDataIqRef_.fSetpoint_  IndexOptions=Index vector (dialog)  Indices=1  OutputSizes=1
  Data Store Write2 : DataStoreWrite  DataStoreName=oPump  DataStoreElements=oPump.oMot_.oOut_.uiCurrentControllerActive_  IndexOptions=Index vector (dialog)  Indices=1  OutputSizes=1
  fSetpoint_ : Outport
  wires:
  Constant1/1 -> Data Store Write2/1
  Constant/1 -> fSetpoint_/1, Data Store Write/1

== system Target_Control_System/Target_Control_System/MainLoop/pumpMotor_mainLoop/motorTaskMainFastStep(&oPump)/Control Loops - Pump/Sim Options Pump OmegaERef Variant Subsystem/Sim Options 0 Pump OmegaE Subsystem ==
  Data Store Read88 : DataStoreRead  DataStoreName=oPump  DataStoreElements=oPump.oMot_.oState_.oRampDataOmegaERef_.fSetpoint_  IndexOptions=Index vector (dialog)  Indices=1  OutputSizes=1
  Out1 : Outport
  wires:
  Data Store Read88/1 -> Out1/1
